simulink model "Narnia_eval_model"  (R2023b)
settings: Solver=VariableStepAuto  StartTime=0.0  StopTime=24  FixedStep=1  MaxStep=0.01  MinStep=0.001  RelTol=1e-3  EnableMultiTasking=on
values from neighbouring files (symbols this model uses):
  P = 0.2    [train_agent.m]
undefined symbols (not defined in the file or in its folder): A, B, C, DiscIntNeverNeededParam, E, HeatLimit
libraries: simulink x4, eeGeneralControl x1, rllib x1
settings Model: Creator=The MathWorks, Inc.  LastModifiedBy=hdt
settings SolverCC: AlgebraicLoopSolver=TrustRegion  MinimalZcImpactIntegration=on
settings DataIOCC: LimitDataPoints=on  SaveFormat=Array
settings OptimizationCC: ReuseModelBlockBuffer=off  LifeSpan=inf
settings DebuggingCC: UnconnectedInputMsg=warning  UnconnectedOutputMsg=warning  UnconnectedLineMsg=warning  SFUnexpectedBacktrackingDiag=warning  SFNoUnconditionalDefaultTransitionDiag=warning  SFExecutionAtInitializationDiag=none  ArithmeticOperatorsInVariantConditions=warning
settings HardwareCC: ProdBitPerPointer=32  ProdBitPerSizeT=32  ProdBitPerPtrDiffT=32  ProdLargestAtomicFloat=None  ProdIntDivRoundTo=Undefined  ProdEndianess=Unspecified  ProdWordSize=32  ProdHWDeviceType=32-bit Generic
settings ModelReferenceCC: EnableRefExpFcnMdlSchedulingChecks=on  PropagateSignalLabelsOutOfModel=off
settings SFSimCC: SimUseLocalCustomCode=off  CustomCodeUndefinedFunction=UseInterfaceOnly
settings RTWCC: RTWUseLocalCustomCode=off
settings CodeAppCC: StateflowObjectComments=on
settings GRTTargetCC: TargetLangStandard=C89/C90 (ANSI)
settings ConfigComp: CovMetricSettings=dw  CovSaveCumulativeToWorkspaceVar=on  CovSaveSingleToWorkspaceVar=on  CovExternalEMLEnable=off  CovSFcnEnable=off

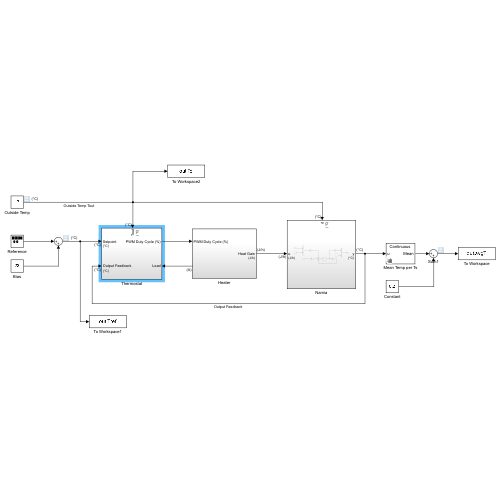
[thumbnail: Simulink's stored preview of the top-level diagram]
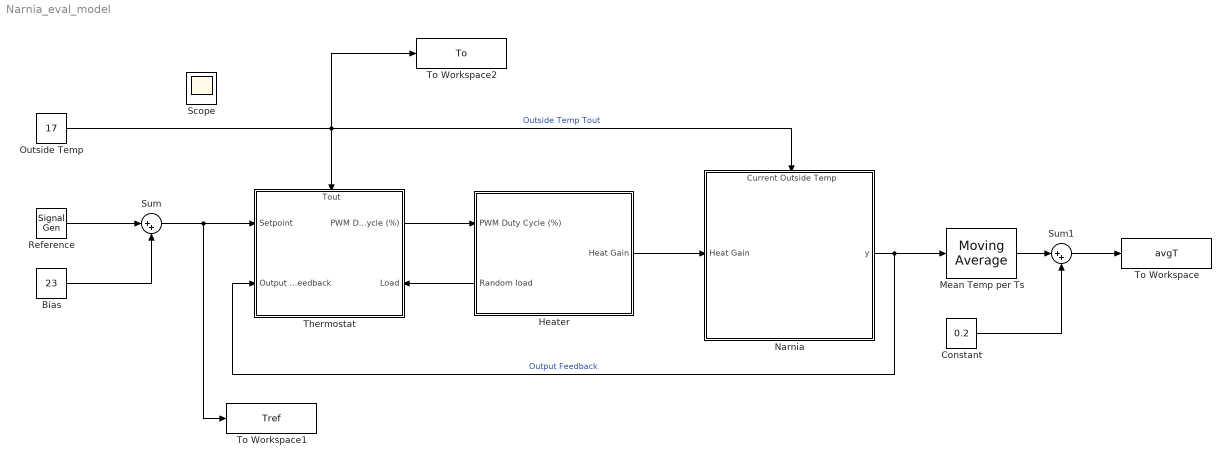
== system Narnia_eval_model ==
  Bias : Constant  Value=23  SampleTime=1
  Constant : Constant  Value=0.2
  Heater : Subsystem
      settings: PortSchema="{\"entries\":[{\"content\":{\"sides\":[{\"content\":{\"connectorIds\":[\"In1\",\"Out2\"]},\"type\":\"ConnectorPlacement.EquallySpacedRectSide\",\"uuid\":\"4f8bdedb-4691-4645-9e5a-9d4cb9ebd4ea\"},{\"content\":{\"connectorIds\":[\"Out1\"],\"side\":\"RIGHT\"},\"type\":\"ConnectorPlacement.EquallySpacedRectSide\",\"uuid\":\"7d395606-f423-4b67-a102-5e58262706c1\"},{\"content\":{\"side\":\"TOP\"},\"type\":\"ConnectorPlacement.EquallySpacedRectSide\",\"uuid\":\"b7d096a7-af21-44a5-847f-d752d23dd21c\"}]},\"type\":\"ConnectorPlacement.EquallySpacedConnector\",\"uuid\":\"6f48db0c-acf9-47d8-b91b-c0b3a1fd4bfd\"}],\"packageUris\":[\"http://schema.mathworks.com/mf0/Connector/R2020b\"],\"version\":\"1.0\"}"
  Mean Temp per Ts : eeGeneralControl/Moving Average  VariantControl=Variant1  LabelModeActiveChoice=Continuous  f=1  x0=11  BufferSize=8192  Ts=0
      settings: LibrarySourceBlock=ee_sl_lib/General Control/Moving Average
  Narnia : Subsystem
      settings: PortSchema="{\"entries\":[{\"content\":{\"sides\":[{\"content\":{\"connectorIds\":[\"In1\"]},\"type\":\"ConnectorPlacement.EquallySpacedRectSide\",\"uuid\":\"190832a2-0d7b-429a-8a42-d587dcc25890\"},{\"content\":{\"connectorIds\":[\"Out1\"],\"side\":\"RIGHT\"},\"type\":\"ConnectorPlacement.EquallySpacedRectSide\",\"uuid\":\"b8632c73-fea3-48b7-a581-c90e1ed24b24\"},{\"content\":{\"connectorIds\":[\"In2\"],\"side\":\"TOP\"},\"type\":\"ConnectorPlacement.EquallySpacedRectSide\",\"uuid\":\"193ecef7-bade-4674-8051-a43898fe5452\"}]},\"type\":\"ConnectorPlacement.EquallySpacedConnector\",\"uuid\":\"7b11e8d5-f5a5-413c-8c1c-b639b4d10c77\"}],\"packageUris\":[\"http://schema.mathworks.com/mf0/Connector/R2020b\"],\"version\":\"1.0\"}"
  Outside Temp : Constant  Value=17
  Reference : SignalGenerator  WaveForm=square  Frequency=pi/4  Units=rad/sec
  Sum : Sum  Inputs=|++
  Sum1 : Sum  Inputs=|++
  Thermostat : Subsystem
      settings: PortSchema="{\"entries\":[{\"content\":{\"sides\":[{\"content\":{\"connectorIds\":[\"In1\",\"In2\"]},\"type\":\"ConnectorPlacement.EquallySpacedRectSide\",\"uuid\":\"895fbc35-389f-4678-9b0a-70c435693bfc\"},{\"content\":{\"connectorIds\":[\"Out1\",\"In4\"],\"side\":\"RIGHT\"},\"type\":\"ConnectorPlacement.EquallySpacedRectSide\",\"uuid\":\"8d167a41-533a-4be9-a4c1-965acf402f2c\"},{\"content\":{\"connectorIds\":[\"In3\"],\"side\":\"TOP\"},\"type\":\"ConnectorPlacement.EquallySpacedRectSide\",\"uuid\":\"c28d814a-5705-450e-be60-09afb29145b8\"},{\"content\":{\"side\":\"BOTTOM\"},\"type\":\"ConnectorPlacement.EquallySpacedRectSide\",\"uuid\":\"e32535bb-66ba-4e7f-9437-3af120630a67\"}]},\"type\":\"ConnectorPlacement.EquallySpacedConnector\",\"uuid\":\"9afdbd54-8878-403f-8397-85eadd1ad1fc\"}],\"packageUris\":[\"http://schema.mathworks.com/mf0/Connector/R2020b\"],\"version\":\"1.0\"}"
  To Workspace : ToWorkspace  VariableName=avgT  SaveFormat=Timeseries  SampleTime=-1
  To Workspace1 : ToWorkspace  VariableName=Tref  SaveFormat=Timeseries  SampleTime=-1
  To Workspace2 : ToWorkspace  VariableName=To  SaveFormat=Timeseries  SampleTime=-1
  Scope : Scope
  wires:
  Thermostat/1(PWM Duty Cycle (%)) -> Heater/1(PWM Duty Cycle (%))
  Heater/1(Heat Gain) -> Narnia/1(Heat Gain)
  Narnia/1(y) -> Mean Temp per Ts/1, Thermostat/2(Output Feedback)  "Output Feedback"
  Sum/1 -> To Workspace1/1, Thermostat/1(Setpoint)
  Mean Temp per Ts/1 -> Sum1/1
  Heater/2(Random load) -> Thermostat/4(Load)
  Outside Temp/1 -> To Workspace2/1, Narnia/2(Current Outside Temp), Thermostat/3(Tout)  "Outside Temp Tout"
  Reference/1 -> Sum/1
  Bias/1 -> Sum/2
  Constant/1 -> Sum1/2
  Sum1/1 -> To Workspace/1

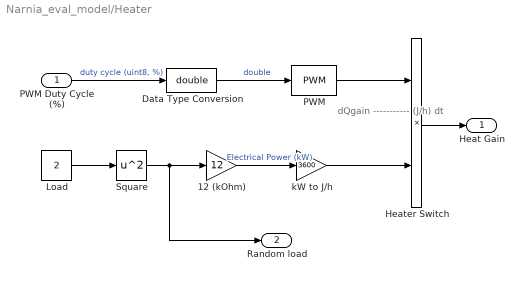
== system Narnia_eval_model/Heater ==
  note: dQgain
      | ----------- (J/h)
      |    dt
  PWM Duty Cycle (%) : Inport
  12 (kOhm) : Gain  Gain=12
  Data Type Conversion : DataTypeConversion  OutDataTypeStr=double  RndMeth=Round  SaturateOnIntegerOverflow=off
  Heater Switch : Product  RndMeth=Zero
  Load : Constant  Value=2
  PWM : simulink/Discontinuities/PWM  DisableCoverage=on  Period=P  InitialDelay=0  DisallowZeroDutyCycle=off  RunAtFixedTimeIntervals=off  SampleTime=0.1
  Square : Math  Operator=square
  kW to J/h : Gain  Gain=3600
  Heat Gain : Outport  Unit=joule/hour  VectorParamsAs1DForOutWhenUnconnected=off
  Random load : Outport  Port=2  Unit=A
  wires:
  PWM/1 -> Heater Switch/1
  Heater Switch/1 -> Heat Gain/1
  kW to J/h/1 -> Heater Switch/2
  Data Type Conversion/1 -> PWM/1  "double"
  PWM Duty Cycle (%)/1 -> Data Type Conversion/1  "duty cycle (uint8, %)"
  12 (kOhm)/1 -> kW to J/h/1  "Electrical Power (kW)"
  Load/1 -> Square/1
  Square/1 -> 12 (kOhm)/1, Random load/1

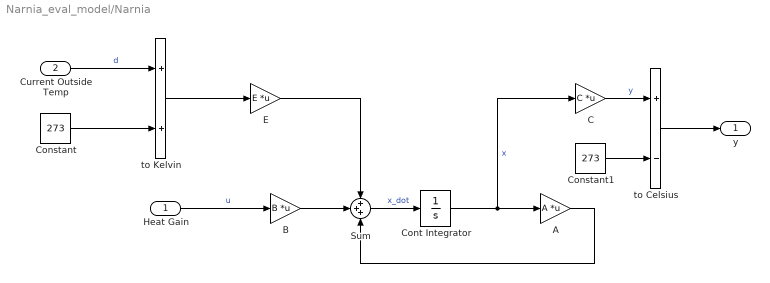
== system Narnia_eval_model/Narnia ==
  Heat Gain : Inport  Unit=J/h
  Current Outside Temp : Inport  Port=2  Unit=Celsius
  A : Gain  Gain=A  Multiplication=Matrix(K*u)
  B : Gain  Gain=B  Multiplication=Matrix(K*u)
  C : Gain  Gain=C  Multiplication=Matrix(K*u)
  Constant : Constant  Value=273
  Constant1 : Constant  Value=273
  Cont Integrator : Integrator  InitialCondition=290
  E : Gain  Gain=E  Multiplication=Matrix(K*u)
  Sum : Sum  Inputs=+++
  to Celsius : Sum  Inputs=+-
  to Kelvin : Sum
  y : Outport  Unit=°C
  wires:
  Heat Gain/1 -> B/1  "u"
  B/1 -> Sum/2
  A/1 -> Sum/3
  Sum/1 -> Cont Integrator/1  "x_dot"
  Cont Integrator/1 -> C/1, A/1  "x"
  E/1 -> Sum/1
  Current Outside Temp/1 -> to Kelvin/1  "d"
  C/1 -> to Celsius/1  "y"
  Constant/1 -> to Kelvin/2
  to Kelvin/1 -> E/1
  to Celsius/1 -> y/1
  Constant1/1 -> to Celsius/2

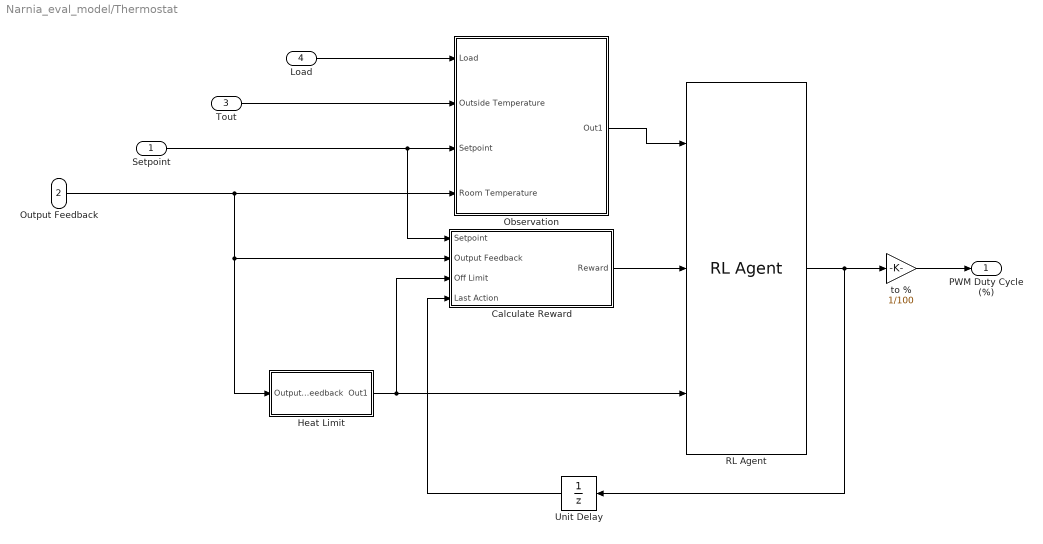
== system Narnia_eval_model/Thermostat ==
  Setpoint : Inport  Unit=°C
  Output Feedback : Inport  Port=2  Unit=°C
  Tout : Inport  Port=3  Unit=°C
  Load : Inport  Port=4
  Calculate Reward : Subsystem
  Heat Limit : Subsystem
  Observation : Subsystem
  RL Agent : rllib/RL Agent  Agent=bl8c_oj_uint8_3k6_lqr  ExternalActionAsInput=off  ProvideLastAction=off  ProvideCumRwd=off  TreatAsDirectFeedthrough=on  UseStrictObservationDataTypes=off
  Unit Delay : UnitDelay  SampleTime=-1  HasFrameUpgradeWarning=on
  to % : Gain  Gain=1/100
  PWM Duty Cycle (%) : Outport  VectorParamsAs1DForOutWhenUnconnected=off
  wires:
  Setpoint/1 -> Calculate Reward/1(Setpoint), Observation/3(Setpoint)
  Output Feedback/1 -> Heat Limit/1(Output Feedback), Calculate Reward/2(Output Feedback), Observation/4("    Room Temperature")
  Tout/1 -> Observation/2(Outside Temperature)
  Observation/1(Out1) -> RL Agent/1
  Calculate Reward/1(Reward) -> RL Agent/2
  Heat Limit/1(Out1) -> Calculate Reward/3(Off Limit), RL Agent/3
  RL Agent/1 -> Unit Delay/1, to %/1
  to %/1 -> PWM Duty Cycle (%)/1
  Unit Delay/1 -> Calculate Reward/4(Last Action)
  Load/1 -> Observation/1(Load)

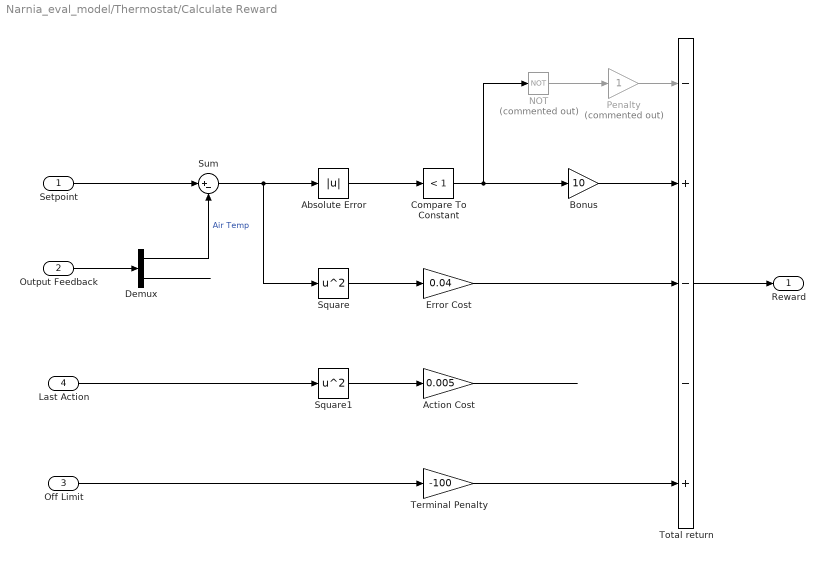
== system Narnia_eval_model/Thermostat/Calculate Reward ==
  Setpoint : Inport
  Output Feedback : Inport  Port=2
  Off Limit : Inport  Port=3
  Last Action : Inport  Port=4
  Absolute Error : Abs  SaturateOnIntegerOverflow=off
  Action Cost : Gain  Gain=0.005
  Bonus : Gain  Gain=10
  Compare To Constant : simulink/Logic and Bit Operations/Compare To Constant  relop=<  const=1  OutDataTypeStr=boolean
  Demux : Demux  Outputs=2
  Error Cost : Gain  Gain=0.04
  NOT : Logic  Commented=on  Operator=NOT  IconShape=distinctive  AllPortsSameDT=off  OutDataTypeStr=boolean
  Penalty : Gain  Commented=on
  Square : Math  Operator=square
  Square1 : Math  Operator=square
  Sum : Sum  Inputs=|+-
  Terminal Penalty : Gain  Gain=-100
  Total return : Sum  Inputs=-+--+
  Reward : Outport
  wires:
  Setpoint/1 -> Sum/1
  Total return/1 -> Reward/1
  Terminal Penalty/1 -> Total return/5
  Off Limit/1 -> Terminal Penalty/1
  Sum/1 -> Square/1, Absolute Error/1
  Output Feedback/1 -> Demux/1
  Absolute Error/1 -> Compare To Constant/1
  Bonus/1 -> Total return/2
  Compare To Constant/1 -> NOT/1, Bonus/1
  Penalty/1 -> Total return/1
  NOT/1 -> Penalty/1
  Demux/1 -> Sum/2  "Air Temp"
  Demux/2 -> ?
  Error Cost/1 -> Total return/3
  Square/1 -> Error Cost/1
  Square1/1 -> Action Cost/1
  Action Cost/1 -> ?
  Last Action/1 -> Square1/1

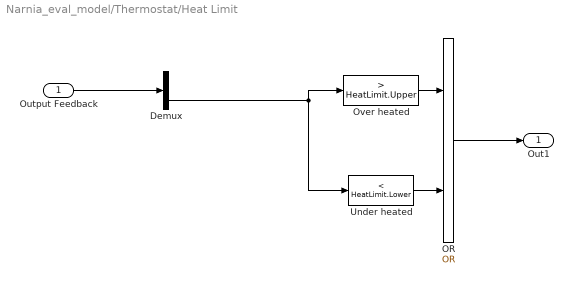
== system Narnia_eval_model/Thermostat/Heat Limit ==
  Output Feedback : Inport
  Demux : Demux  Outputs=2
  OR : Logic  Operator=OR  IconShape=distinctive  AllPortsSameDT=off  OutDataTypeStr=boolean
  Over heated : simulink/Logic and Bit Operations/Compare To Constant  relop=>  const=HeatLimit.Upper  OutDataTypeStr=boolean
  Under heated : simulink/Logic and Bit Operations/Compare To Constant  relop=<  const=HeatLimit.Lower  OutDataTypeStr=boolean
  Out1 : Outport
  wires:
  Demux/2 -> Under heated/1, Over heated/1
  Under heated/1 -> OR/2
  Over heated/1 -> OR/1
  OR/1 -> Out1/1
  Output Feedback/1 -> Demux/1

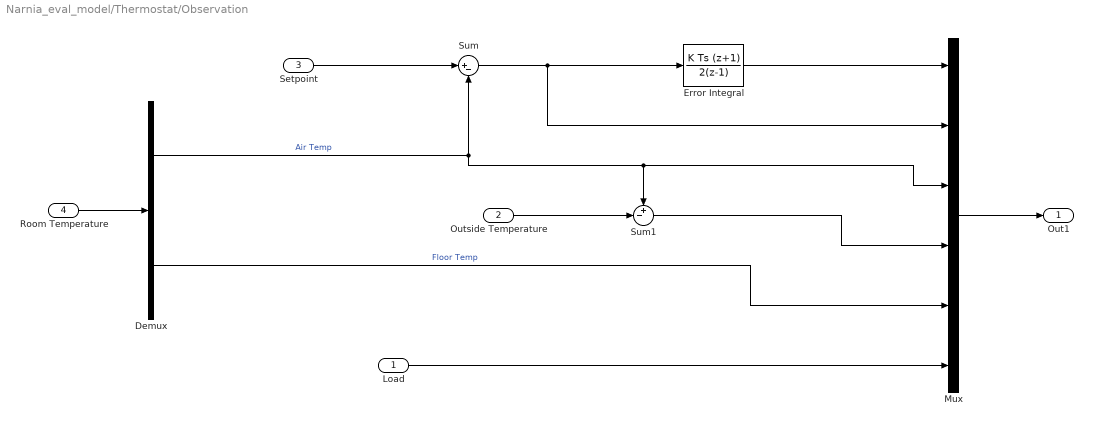
== system Narnia_eval_model/Thermostat/Observation ==
  Load : Inport
  Outside Temperature : Inport  Port=2
  Setpoint : Inport  Port=3
  "    Room Temperature" : Inport  Port=4
  Demux : Demux  Outputs=2
  Error Integral : DiscreteIntegrator  IntegratorMethod=Integration: Trapezoidal  SampleTime=-1  ICPrevOutput=DiscIntNeverNeededParam  ICPrevScaledInput=DiscIntNeverNeededParam
  Mux : Mux  Inputs=6
  Sum : Sum  Inputs=|+-
  Sum1 : Sum  Inputs=+-|
  Out1 : Outport
  wires:
  Setpoint/1 -> Sum/1
  Demux/1 -> Sum1/1, Mux/3, Sum/2  "Air Temp"
  Error Integral/1 -> Mux/1
  Mux/1 -> Out1/1
  Sum/1 -> Error Integral/1, Mux/2
  "    Room Temperature"/1 -> Demux/1
  Demux/2 -> Mux/5  "Floor Temp"
  Load/1 -> Mux/6
  Sum1/1 -> Mux/4
  Outside Temperature/1 -> Sum1/2
